simulink model "main"  (R2023b)
settings: Solver=ode4  StartTime=0.0  StopTime=20  FixedStep=0.0001  RelTol=1e-3  AbsTol=1e-3  EnableMultiTasking=on
undefined symbols (not defined in the file or in its folder): X, Y, Z
libraries: sm_lib x85, nesl_utility x19, simulink_extras x4, ArmLibrary x2, gripper_v2_bottom x2, gripper_v2_top x2, lower_link_v2 x1, WorkSpaceLibrarry x1
(part 2 of 2)

== matlab function main/MATLAB Function ==
  data: t input; y output; p input
function y = fcn(t, p) 
    % ===================================================================== 
    % CONTROL PARAMETERS 
    % ===================================================================== 
    F_clamp             = -400;    % Target full clamping force (N) 
     
    % --- Initial Clamping Parameters --- 
    F_approach1         = -1;     % Gentle approach force for first clamp (N) 
    p_stiffness1        = 0.002;    % Penetration depth for full force (m) 
     
    % --- Second Clamping Parameters (Specific to final phase) --- 
    F_approach_clamp2   = -0.001;     % Gentle approach force for second clamp (N) 
    p_stiffness_clamp2  = 0.0015;   % Penetration depth for second clamp (m) 
     
    p_contact           = 0.0;      % Contact position threshold (m) 
     
    p_start             = -0.015;   % Position when clamped (m) 
    p_target            = -15e-3;     % Target release position (m) 
     
    t_release           = 0.5;      % Time to start release (s) 
    move_dur            = 0.8;      % Duration of release movement (s) 
     
    Kp                  = 150;      % Position tracking gain (N/m) 
    Kd_scale            = 0.5;      % Braking scale when overshooting 
     
    t_second_clamp      = 16.5;      % Time to re-engage clamping (s) 
    % ===================================================================== 
    p_start2 = 0.06; 
    p_target2 =0; 
     
    % 1. Initial Clamping Phase 
    if t < t_release 
        if p < p_contact 
            % Gentle approach before contact 
            y = F_approach1; 
        else 
            % Smooth force ramp upon contact based on deflection 
            contact_ratio = min(1.0, (p - p_contact) / p_stiffness1); 
            y = F_approach1 + (F_clamp - F_approach1) * contact_ratio; 
        end 
         
    % 2. S-Curve Release & Dynamic Hold Phase 
    elseif t >= t_release && t < (t_second_clamp-1.5) 
        tau = min(1.0, (t - t_release) / move_dur); 
         
        s_curve = tau^3 * (6 * tau^2 - 15 * tau + 10); 
        p_ref = p_start + (p_target - p_start) * s_curve; 
         
        err = p_ref - p; 
        p_start2=p; 
        if err >= 0 
            y = Kp * err; 
        else 
            y = Kp * err * (1 + Kd_scale * abs(err)); 
        end 
         
        if tau >= 1.0 
            if abs(p_target - p) < 0.003 
                y = y * (abs(p_target - p) / 0.003); 
            end 
        end 
         
    % 3. Second Clamping Phase (t >= t_second_clamp) 
    elseif t > (t_second_clamp-1.5)  && t <t_second_clamp 
        tau = min(1.0, (t - (t_second_clamp-1.5)) / move_dur); 
         
        s_curve = tau^3 * (6 * tau^2 - 15 * tau + 10); 
        p_ref = p_start2 + (p_target2 - p_start2) * s_curve; 
         
        err = p_ref - p; 
         
        if err >= 0 
            y = Kp * err; 
        else 
            y = Kp * err * (1 + Kd_scale * abs(err)); 
        end 
         
        if tau >= 1.0 
            if abs(p_target2 - p) < 0.003 
                y = y * (abs(p_target2 - p) / 0.003); 
            end 
        end 
    else 
        y = -500; 
    end 
end

== matlab function main/MATLAB Function2 ==
  data: t input; y output

function y = angle2(t)

    % Each row represents one motion:
    % [t_start, duration, y_start, y_end]

    movements = [
      
        1.5, 1.0,   0,   -6;
        5.5, 4.0,   -6,   186;

    ];

    % Initial position
    y = movements(1,3);

    % Check each movement
    for i = 1:size(movements,1)

        t_start = movements(i,1);
        duration = movements(i,2);
        y_start = movements(i,3);
        y_end = movements(i,4);

        if t <= t_start

            % Before movement starts
            y = y_start;
            return

        elseif t < (t_start + duration)

            % During movement
            tau = (t - t_start) / duration;

            % 5th-order smooth trajectory
            s = 6*tau^5 - 15*tau^4 + 10*tau^3;

            y = y_start + (y_end - y_start) * s;
            return

        else

            % Movement completed
            y = y_end;

        end
    end
end

== matlab function main/MATLAB Function3 ==
  data: t input; y output
function y = angle(t)
    t_start = 2.5;    % Time when movement begins
    duration = 0.5;   % Transition time in seconds (increase if still too fast)
    
    y_start = 0+115;
    y_end   = -10+115;
    
    if t <= t_start
        y = y_start;
    elseif t >= (t_start + duration)
        y = y_end;
    else
        % Normalized time normalized between 0 and 1
        tau = (t - t_start) / duration;
        
        % 5th-order polynomial (smooth 1st and 2nd derivatives)
        s = 6*tau^5 - 15*tau^4 + 10*tau^3;
        
        y = y_start + (y_end - y_start) * s;
    end
end

== matlab function main/MATLAB Function4 ==
  data: t input; y output
function y = angle(t)

    % Each row represents one movement:
    % [t_start, duration, y_start, y_end]

    movements = [
        3.0, 0.5,   -90-25.5,   -90;
      
    ];

    % Default value
    y = movements(1,3);

    % Check each movement
    for i = 1:size(movements,1)

        t_start = movements(i,1);
        duration = movements(i,2);
        y_start = movements(i,3);
        y_end = movements(i,4);

        if t <= t_start
            y = y_start;
            return

        elseif t < (t_start + duration)

            % Normalized time
            tau = (t - t_start) / duration;

            % 5th-order smooth polynomial
            s = 6*tau^5 - 15*tau^4 + 10*tau^3;

            y = y_start + (y_end - y_start) * s;
            return

        else
            % Movement is complete
            y = y_end;
        end
    end
end
